simulink subsystem "IMU"  (R2024b)
settings: Solver=VariableStepAuto  StartTime=0.0  StopTime=10.0  RelTol=1e-3
undefined symbols (not defined in the file): dt
libraries: raspberrypiCommlib x14
settings Model: Creator=schwmaxi  LastModifiedBy=schwmaxi

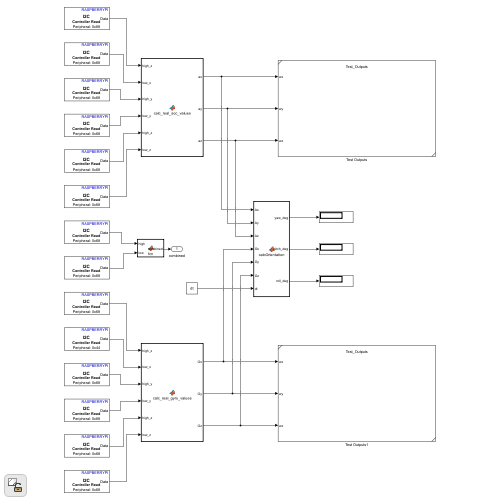
[thumbnail: Simulink's stored preview of the top-level diagram]
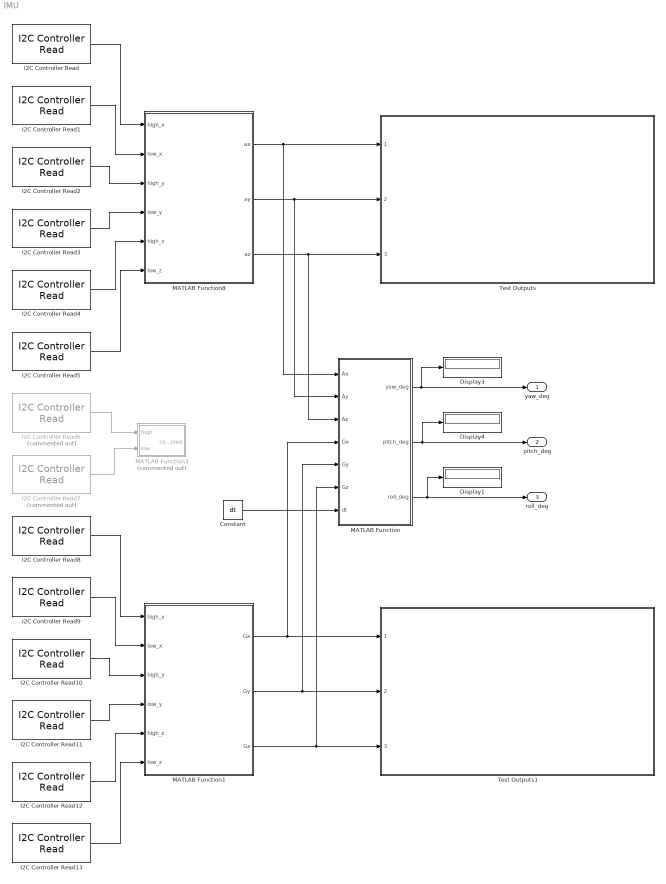
== system IMU ==
  Constant : Constant  Value=dt
  Display1 : Display
  Display3 : Display
  Display4 : Display
  I2C Controller Read : raspberrypiCommlib/I2C Controller Read  BoardProperty=Pi 4 Model B  I2CModule=1  Mode=Master  SlaveAddress=0x68  SlaveByteOrder=BigEndian  Direction=Receiver  RegisterAddressMode=on  RegisterAddress=0x3B  SlaveDataType=uint8  DataLength=1  NoAck=off  RepeatedStart=off  OutputStatus=off  SampleTime=0.1
  I2C Controller Read1 : raspberrypiCommlib/I2C Controller Read  BoardProperty=Pi 4 Model B  I2CModule=1  Mode=Master  SlaveAddress=0x68  SlaveByteOrder=BigEndian  Direction=Receiver  RegisterAddressMode=on  RegisterAddress=0x3C  SlaveDataType=uint8  DataLength=1  NoAck=off  RepeatedStart=off  OutputStatus=off  SampleTime=0.1
  I2C Controller Read10 : raspberrypiCommlib/I2C Controller Read  BoardProperty=Pi 4 Model B  I2CModule=1  Mode=Master  SlaveAddress=0x68  SlaveByteOrder=BigEndian  Direction=Receiver  RegisterAddressMode=on  RegisterAddress=0x45  SlaveDataType=uint8  DataLength=1  NoAck=off  RepeatedStart=off  OutputStatus=off  SampleTime=0.1
  I2C Controller Read11 : raspberrypiCommlib/I2C Controller Read  BoardProperty=Pi 4 Model B  I2CModule=1  Mode=Master  SlaveAddress=0x68  SlaveByteOrder=BigEndian  Direction=Receiver  RegisterAddressMode=on  RegisterAddress=0x46  SlaveDataType=uint8  DataLength=1  NoAck=off  RepeatedStart=off  OutputStatus=off  SampleTime=0.1
  I2C Controller Read12 : raspberrypiCommlib/I2C Controller Read  BoardProperty=Pi 4 Model B  I2CModule=1  Mode=Master  SlaveAddress=0x68  SlaveByteOrder=BigEndian  Direction=Receiver  RegisterAddressMode=on  RegisterAddress=0x47  SlaveDataType=uint8  DataLength=1  NoAck=off  RepeatedStart=off  OutputStatus=off  SampleTime=0.1
  I2C Controller Read13 : raspberrypiCommlib/I2C Controller Read  BoardProperty=Pi 4 Model B  I2CModule=1  Mode=Master  SlaveAddress=0x68  SlaveByteOrder=BigEndian  Direction=Receiver  RegisterAddressMode=on  RegisterAddress=0x48  SlaveDataType=uint8  DataLength=1  NoAck=off  RepeatedStart=off  OutputStatus=off  SampleTime=0.1
  I2C Controller Read2 : raspberrypiCommlib/I2C Controller Read  BoardProperty=Pi 4 Model B  I2CModule=1  Mode=Master  SlaveAddress=0x68  SlaveByteOrder=BigEndian  Direction=Receiver  RegisterAddressMode=on  RegisterAddress=0x3D  SlaveDataType=uint8  DataLength=1  NoAck=off  RepeatedStart=off  OutputStatus=off  SampleTime=0.1
  I2C Controller Read3 : raspberrypiCommlib/I2C Controller Read  BoardProperty=Pi 4 Model B  I2CModule=1  Mode=Master  SlaveAddress=0x68  SlaveByteOrder=BigEndian  Direction=Receiver  RegisterAddressMode=on  RegisterAddress=0x3E  SlaveDataType=uint8  DataLength=1  NoAck=off  RepeatedStart=off  OutputStatus=off  SampleTime=0.1
  I2C Controller Read4 : raspberrypiCommlib/I2C Controller Read  BoardProperty=Pi 4 Model B  I2CModule=1  Mode=Master  SlaveAddress=0x68  SlaveByteOrder=BigEndian  Direction=Receiver  RegisterAddressMode=on  RegisterAddress=0x3F  SlaveDataType=uint8  DataLength=1  NoAck=off  RepeatedStart=off  OutputStatus=off  SampleTime=0.1
  I2C Controller Read5 : raspberrypiCommlib/I2C Controller Read  BoardProperty=Pi 4 Model B  I2CModule=1  Mode=Master  SlaveAddress=0x68  SlaveByteOrder=BigEndian  Direction=Receiver  RegisterAddressMode=on  RegisterAddress=0x40  SlaveDataType=uint8  DataLength=1  NoAck=off  RepeatedStart=off  OutputStatus=off  SampleTime=0.1
  I2C Controller Read6 : raspberrypiCommlib/I2C Controller Read  Commented=on  BoardProperty=Pi 4 Model B  I2CModule=1  Mode=Master  SlaveAddress=0x68  SlaveByteOrder=BigEndian  Direction=Receiver  RegisterAddressMode=on  RegisterAddress=0x41  SlaveDataType=uint8  DataLength=1  NoAck=off  RepeatedStart=off  OutputStatus=off  SampleTime=0.1
  I2C Controller Read7 : raspberrypiCommlib/I2C Controller Read  Commented=on  BoardProperty=Pi 4 Model B  I2CModule=1  Mode=Master  SlaveAddress=0x68  SlaveByteOrder=BigEndian  Direction=Receiver  RegisterAddressMode=on  RegisterAddress=0x42  SlaveDataType=uint8  DataLength=1  NoAck=off  RepeatedStart=off  OutputStatus=off  SampleTime=0.1
  I2C Controller Read8 : raspberrypiCommlib/I2C Controller Read  BoardProperty=Pi 4 Model B  I2CModule=1  Mode=Master  SlaveAddress=0x68  SlaveByteOrder=BigEndian  Direction=Receiver  RegisterAddressMode=on  RegisterAddress=0x43  SlaveDataType=uint8  DataLength=1  NoAck=off  RepeatedStart=off  OutputStatus=off  SampleTime=0.1
  I2C Controller Read9 : raspberrypiCommlib/I2C Controller Read  BoardProperty=Pi 4 Model B  I2CModule=1  Mode=Master  SlaveAddress=0x44  SlaveByteOrder=BigEndian  Direction=Receiver  RegisterAddressMode=on  RegisterAddress=0x3C  SlaveDataType=uint8  DataLength=1  NoAck=off  RepeatedStart=off  OutputStatus=off  SampleTime=0.1
  MATLAB Function : MATLAB Function  TreatAsAtomicUnit=on
  MATLAB Function1 : MATLAB Function  TreatAsAtomicUnit=on
  MATLAB Function3 : MATLAB Function  Commented=on  TreatAsAtomicUnit=on
  MATLAB Function8 : MATLAB Function  TreatAsAtomicUnit=on
  Test Outputs : Subsystem  ReferencedSubsystem=Test_Outputs
  Test Outputs1 : Subsystem  ReferencedSubsystem=Test_Outputs
  yaw_deg : Outport
  pitch_deg : Outport  Port=2
  roll_deg : Outport  Port=3
  wires:
  MATLAB Function1/1(Gx) -> MATLAB Function/4(Gx), Test Outputs1/1
  MATLAB Function/2(pitch_deg) -> Display4/1, pitch_deg/1
  MATLAB Function/3(roll_deg) -> roll_deg/1, Display1/1
  I2C Controller Read6/1 -> MATLAB Function3/1(high)
  I2C Controller Read8/1 -> MATLAB Function1/1(high_x)
  I2C Controller Read12/1 -> MATLAB Function1/5(high_z)
  I2C Controller Read/1 -> MATLAB Function8/1(high_x)
  MATLAB Function1/3(Gz) -> Test Outputs1/3, MATLAB Function/6(Gz)
  MATLAB Function8/1(ax) -> Test Outputs/1, MATLAB Function/1(Ax)
  I2C Controller Read2/1 -> MATLAB Function8/3(high_y)
  I2C Controller Read1/1 -> MATLAB Function8/2(low_x)
  I2C Controller Read10/1 -> MATLAB Function1/3(high_y)
  I2C Controller Read13/1 -> MATLAB Function1/6(low_z)
  I2C Controller Read11/1 -> MATLAB Function1/4(low_y)
  I2C Controller Read5/1 -> MATLAB Function8/6(low_z)
  Constant/1 -> MATLAB Function/7(dt)
  I2C Controller Read4/1 -> MATLAB Function8/5(high_z)
  MATLAB Function8/2(ay) -> Test Outputs/2, MATLAB Function/2(Ay)
  MATLAB Function8/3(az) -> MATLAB Function/3(Az), Test Outputs/3
  I2C Controller Read9/1 -> MATLAB Function1/2(low_x)
  I2C Controller Read3/1 -> MATLAB Function8/4(low_y)
  I2C Controller Read7/1 -> MATLAB Function3/2(low)
  MATLAB Function1/2(Gy) -> MATLAB Function/5(Gy), Test Outputs1/2
  MATLAB Function/1(yaw_deg) -> Display3/1, yaw_deg/1

== matlab function IMU/MATLAB Function1 ==
  data: high_x input; Gx output; Gy output; Gz output; low_x input; high_y input; low_y input; high_z input; low_z input
function [Gx, Gy, Gz] = calc_real_gyro_values(high_x, low_x, high_y, low_y, high_z, low_z)
    Gx = double(0.0);
    Gy = double(0.0);
    Gz = double(0.0);

    Gx = combine(high_x, low_x) / 131.0;
    Gy = combine(high_y, low_y) / 131.0 + 0.63;
    Gz = combine(high_z, low_z) / 131.0 - 0.34;


function [value] = combine(high_byte, low_byte)
    combined = bitor(bitshift(uint16(high_byte), 8), uint16(low_byte));

    value = double(typecast(combined, 'int16'));

== matlab function IMU/MATLAB Function ==
  data: yaw_deg output; pitch_deg output; roll_deg output; Ax input; Ay input; Az input; Gx input; Gy input; Gz input; dt input
function [yaw_deg, pitch_deg, roll_deg] = calcOrientation(Ax, Ay, Az, Gx, Gy, Gz, dt)
%#codegen

alpha = 0.85; % Complementary filter coefficient

% ---- Persistent variables for integration ----
persistent roll pitch yaw
if isempty(roll), roll = 0; end
if isempty(pitch), pitch = 0; end
if isempty(yaw), yaw = 0; end

% ---- Accelerometer angles ----
acc_roll  = atan2(Ay, Az);
acc_pitch = atan2(-Ax, sqrt(Ay^2 + Az^2));

% ---- Integrate gyro rates ----
% Note: Gx, Gy, Gz in radians/sec
roll  = alpha * (roll  + Gx * dt) + (1 - alpha) * acc_roll;
pitch = alpha * (pitch + Gy * dt) + (1 - alpha) * acc_pitch;
yaw   = yaw + Gz * dt;  % No correction without magnetometer

% ---- Convert to degrees ----
roll_deg  = roll  * (180/pi);
pitch_deg = pitch * (180/pi);
yaw_deg   = yaw   * (180/pi);
end

== matlab function IMU/MATLAB Function3 ==
  data: high input; combined output; low input
function combined = fcn(high, low)

combined = bitor(bitshift(uint16(high), 8), uint16(low));

== matlab function IMU/MATLAB Function8 ==
  data: high_x input; ax output; ay output; az output; low_x input; high_y input; low_y input; high_z input; low_z input
function [ax, ay, az] = calc_real_acc_values(high_x, low_x, high_y, low_y, high_z, low_z)
    ax = double(0.0);
    ay = double(0.0);
    az = double(0.0);

    ax = combine(high_x, low_x) / 16384.0 - 0.01;
    ay = combine(high_y, low_y) / 16384.0 - 0.03;
    az = combine(high_z, low_z) / 16384.0 - 0.05;


function [value] = combine(high_byte, low_byte)
    combined = bitor(bitshift(uint16(high_byte), 8), uint16(low_byte));

    value = double(typecast(combined, 'int16'));
